simulink model "Calculo_Potencia_Instantanea"  (R2014a)
settings: Solver=ode45  StartTime=0.0  StopTime=0.033  MaxStep=1e-4  RelTol=1e-3
libraries: powerlib x3
settings Model: Creator=Joao  LastModifiedBy=Joao

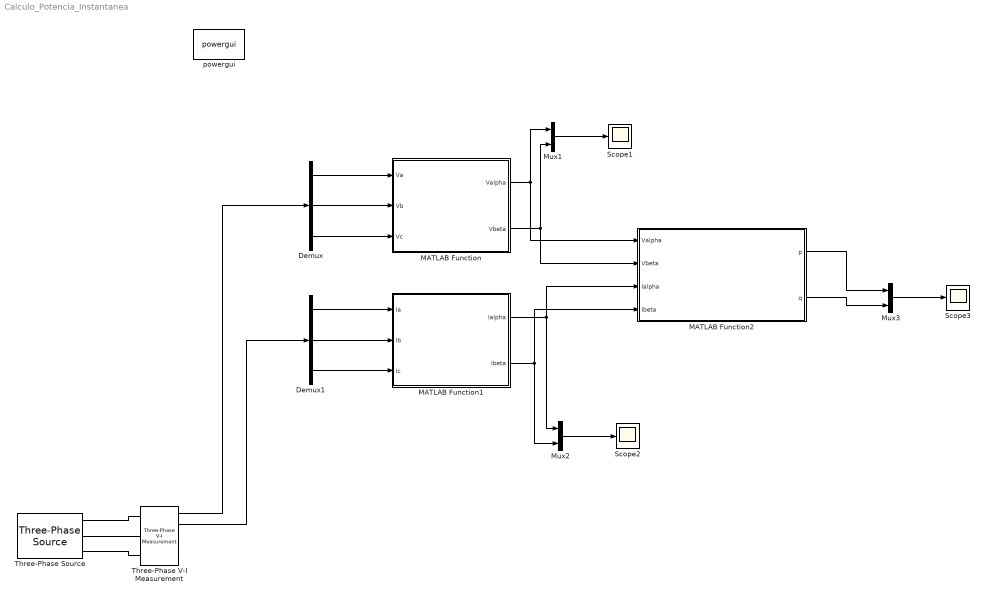
== system Calculo_Potencia_Instantanea ==
  Demux : Demux  Outputs=3
  Demux1 : Demux  Outputs=3
  MATLAB Function : MATLAB Function  TreatAsAtomicUnit=on
  MATLAB Function1 : MATLAB Function  TreatAsAtomicUnit=on
  MATLAB Function2 : MATLAB Function  TreatAsAtomicUnit=on
  Mux1 : Mux  Inputs=2
  Mux2 : Mux  Inputs=2
  Mux3 : Mux  Inputs=2
  Scope1 : Scope
  Scope2 : Scope
  Scope3 : Scope
      settings: SaveName=ScopeData2
  Three-Phase V-I Measurement : powerlib/Measurements/Three-Phase V-I Measurement  VoltageMeasurement=phase-to-ground  SetLabelV=off  LabelV=Vabc  Vpu=off  VpuLL=off  CurrentMeasurement=yes  SetLabelI=off  LabelI=Iabc  Ipu=off  Pbase=100e6  Vbase=500e3  OutputType=Complex  PhasorSimulation=off  PSBequivalent=0
  Three-Phase Source : powerlib/Electrical Sources/Three-Phase Source  Voltage=115  PhaseAngle=0  Frequency=400  InternalConnection=Yg  SpecifyImpedance=on  Resistance=0.8929  Inductance=16.58e-3  ShortCircuitLevel=100e6  BaseVoltage=25e3  XRratio=7  BusType=swing  Pref=0  Qref=0  Qmin=-inf  Qmax=inf
  powergui : powerlib/powergui  Priority=1  SimulationMode=Continuous  SolverType=Tustin  SampleTime=50e-6  frequency=60  SPID=off  DisableSnubberDevices=off  DisableRonSwitches=off  DisableVfSwitches=off  SwTol=0  Interpol=off  DisplayEquations=off  Ts=0  methode=off  frequencyindice=400  Pbase=100e6  ErrMax=1e-4  Iterations=50  UnitsV=kV  UnitsW=MW  FunctionMessages=off  echomessages=off  HookPort=off  EnableUseOfTLC=off  x0status=blocks  RestoreLinks=warning  ResistiveCurrentMeasurement=off  Frange=[0:2:500]  Ylog=off  Xlog=on  ShowGrid=off  save=off  variable=ZData  structure=0  ZoomFFT=off  StartTime=0.0  cycles=1  DisplayStyle=1  fundamental=60  FreqAxis=off  MaxFrequency=1000  frequencyindicesteady=1  RmsSteady=1  display=off
  wires:
  Mux1/1 -> Scope1/1
  Mux2/1 -> Scope2/1
  MATLAB Function/1(Valpha) -> MATLAB Function2/1(Valpha), Mux1/1
  MATLAB Function/2(Vbeta) -> Mux1/2, MATLAB Function2/2(Vbeta)
  MATLAB Function1/1(Ialpha) -> Mux2/1, MATLAB Function2/3(Ialpha)
  MATLAB Function1/2(Ibeta) -> MATLAB Function2/4(Ibeta), Mux2/2
  Demux/3 -> MATLAB Function/3(Vc)
  Demux1/1 -> MATLAB Function1/1(Ia)
  Three-Phase V-I Measurement/1 -> Demux/1
  Three-Phase V-I Measurement/2 -> Demux1/1
  Demux1/2 -> MATLAB Function1/2(Ib)
  Demux1/3 -> MATLAB Function1/3(Ic)
  Demux/1 -> MATLAB Function/1(Va)
  Demux/2 -> MATLAB Function/2(Vb)
  Mux3/1 -> Scope3/1
  MATLAB Function2/1(p) -> Mux3/1
  MATLAB Function2/2(q) -> Mux3/2
  connections:
  Three-Phase Source/RConn1 -- Three-Phase V-I Measurement/LConn1
  Three-Phase Source/RConn2 -- Three-Phase V-I Measurement/LConn2
  Three-Phase Source/RConn3 -- Three-Phase V-I Measurement/LConn3

== matlab function Calculo_Potencia_Instantanea/MATLAB Function1 ==
  data: Ia input; Ialpha output; Ib input; Ic input; Ibeta output
function [Ialpha,Ibeta] = Transformada_Clarke_Corrente(Ia,Ib,Ic)
%#codegen
I = sqrt(2/3)*[1 -1/2 -1/2; 0 sqrt(3)/2 -sqrt(3)/2]*[Ia;Ib;Ic];
Ialpha = I(1,:);
Ibeta = I(2,:);

== matlab function Calculo_Potencia_Instantanea/MATLAB Function ==
  data: Va input; Valpha output; Vb input; Vc input; Vbeta output
function [Valpha,Vbeta] = Transformada_Clarke_Tensao(Va,Vb,Vc)
%#codegen
V = sqrt(2/3)*[1 -1/2 -1/2; 0 sqrt(3)/2 -sqrt(3)/2]*[Va;Vb;Vc];
Valpha = V(1,:);
Vbeta = V(2,:);

== matlab function Calculo_Potencia_Instantanea/MATLAB Function2 ==
  data: Valpha input; Vbeta input; Ialpha input; Ibeta input; p output; q output
function [p,q] = Calculo_Potencia_Instantanea(Valpha,Vbeta,Ialpha,Ibeta)
%#codegen
p = Valpha*Ialpha+Vbeta*Ibeta;
q = Vbeta*Ialpha-Valpha*Ibeta;
